simulink model "solarpanel"  (R2023a)
settings: Solver=VariableStepAuto  StartTime=0.0  StopTime=15*3600  RelTol=1e-3
values from neighbouring files (symbols this model uses):
  J = 8.6    [solarpanel.mat]
  Kd = 5    [solarpanel.mat]
  Kf = 0.07    [solarpanel.mat]
  Kg = 2000    [solarpanel.mat]
  Kt = 0.07    [solarpanel.mat]
  L = 1e-05    [solarpanel.mat]
  R = 10    [solarpanel.mat]
libraries: slpidlib x1
settings Model: Creator=brian  LastModifiedBy=brian
settings DataIOCC: ExternalInput=[sunTime sunPosition]  LoadExternalInput=on

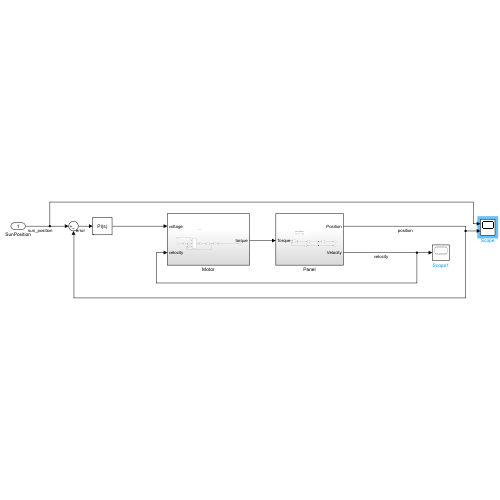
[thumbnail: Simulink's stored preview of the top-level diagram]
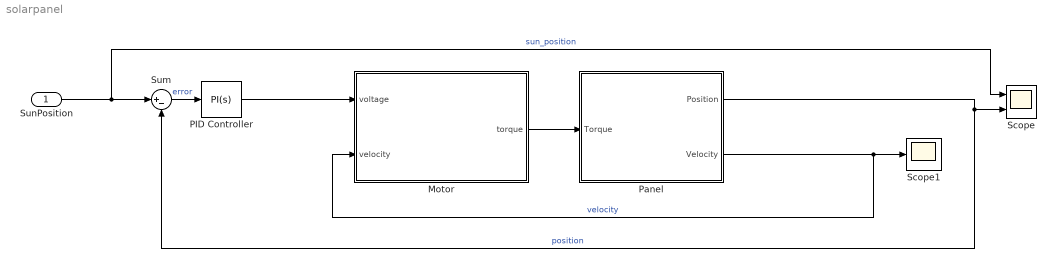
== system solarpanel ==
  SunPosition : Inport
  Motor : Subsystem
  PID Controller : slpidlib/PID Controller  Controller=PI  Form=Parallel  TimeDomain=Continuous-time  UseExternalTs=off  SampleTime=-1  IntegratorMethod=Forward Euler  FilterMethod=Forward Euler  ControllerParametersSource=internal  P=240  I=180  UseKiTs=off  D=0  N=100  UseFilter=on  TunerSelectOption=Transfer Function Based (PID Tuner App)  InitialConditionSource=internal  InitialConditionForIntegrator=0  InitialConditionForFilter=0  DifferentiatorICPrevScaledInput=0  ExternalReset=none  TrackingMode=off  Kt=1  LimitOutput=off  SatLimitsSource=internal  UpperSaturationLimit=inf  LowerSaturationLimit=-inf  LinearizeAsGain=on  AntiWindupMode=none  Kb=1  LimitIntegrator=off  UpperIntegratorSaturationLimit=inf  LowerIntegratorSaturationLimit=-inf  POutMin=[]  POutMax=[]  IOutMin=[]  IOutMax=[]  DOutMin=[]  DOutMax=[]  NOutMin=[]  NOutMax=[]  SumOutMin=[]  SumOutMax=[]  SaturationOutMin=[]  SaturationOutMax=[]  PParamMin=[]  PParamMax=[]  IParamMin=[]  IParamMax=[]  DParamMin=[]  DParamMax=[]  NParamMin=[]  NParamMax=[]  KbParamMin=[]  KbParamMax=[]  KtParamMin=[]  KtParamMax=[]  KbOutMin=[]  KbOutMax=[]  KtOutMin=[]  KtOutMax=[]  IntegratorOutMin=[]  IntegratorOutMax=[]  FilterOutMin=[]  FilterOutMax=[]  SumI1OutMin=[]  SumI1OutMax=[]  SumI2OutMin=[]  SumI2OutMax=[]  SumI3OutMin=[]  SumI3OutMax=[]  SumI4OutMin=[]  SumI4OutMax=[]  SumDOutMin=[]  SumDOutMax=[]  DifferentiatorOutMin=[]  DifferentiatorOutMax=[]  FilterDiffOutCoefMin=[]  FilterDiffOutCoefMax=[]  ReciprocalOutMin=[]  ReciprocalOutMax=[]  SumDenOutMin=[]  SumDenOutMax=[]  SumNumOutMin=[]  SumNumOutMax=[]  DivideOutMin=[]  DivideOutMax=[]  UdiffTsProdOutMin=[]  UdiffTsProdOutMax=[]  NTsProdOutMin=[]  NTsProdOutMax=[]  UintegralTsProdOutMin=[]  UintegralTsProdOutMax=[]  UngainTsProdOutMin=[]  UngainTsProdOutMax=[]  ClampingZeroOutDataTypeStr=Inherit: Inherit via back propagation  ClampingZeroOutMin=[]  ClampingZeroOutMax=[]  FilterDenConstantOutDataTypeStr=Inherit: Inherit via back propagation  FilterDenConstantOutMin=[]  FilterDenConstantOutMax=[]  PCopyOutDataTypeStr=Inherit: Inherit via back propagation  PCopyOutMin=[]  PCopyOutMax=[]  NCopyOutDataTypeStr=Inherit: Inherit via back propagation  NCopyOutMin=[]  NCopyOutMax=[]  IntegratorContinuousStateAttributes=''  IntegratorStateMustResolveToSignalObject=off  IntegratorRTWStateStorageClass=Auto  FilterContinuousStateAttributes=''  FilterStateMustResolveToSignalObject=off  FilterRTWStateStorageClass=Auto  ParallelPVariant=InternalParameters  IdealPVariant=Disabled  IVariant=InternalParameters  DVariant=Disabled  IntegratorVariant=Continuous  SatVariant=Disabled  AWVariant=Passthrough  PCopyVariant=Disabled  TRVariant=Disabled  FdbkBlocksVariant=Forward  IdealPFdbkVariant=Disabled  SatFdbkVariant=Disabled  DerivativeFilterVariant=Disabled  NVariant=Disabled  NCopyVariant=Disabled_SignalSpec  FilterICVariant=Disabled  IntegratorICVariant=InternalICs  ExternalResetVariant=Disabled  TRSumVariant=Passthrough  SumFdbkVariant=Disabled  SumVariant=Sum_PI  TsampFilterVariant=InternalTs  TsampNgainVariant=Passthrough  TsampIntegralVariant=Disabled_SignalSpec  ExternalSaturationOutDataTypeStr=Inherit: Same as second input
  Panel : Subsystem
  Scope : Scope  NumInputPorts=2
  Scope1 : Scope
  Sum : Sum  Inputs=|+-
  wires:
  Panel/1(Position) -> Sum/2, Scope/2  "position"
  Panel/2(Velocity) -> Motor/2(velocity), Scope1/1  "velocity"
  Motor/1(torque) -> Panel/1(Torque)
  PID Controller/1 -> Motor/1(voltage)
  SunPosition/1 -> Scope/1, Sum/1  "sun_position"
  Sum/1 -> PID Controller/1  "error"

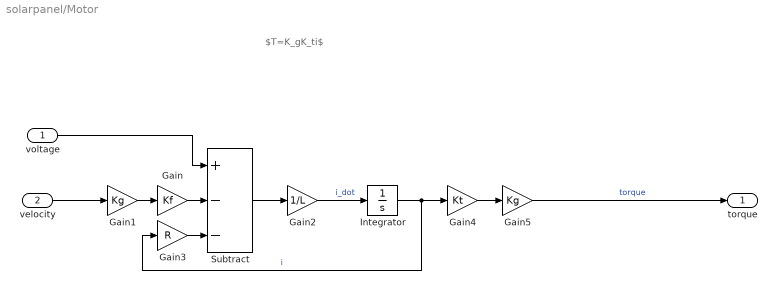
== system solarpanel/Motor ==
  note: $T=K_gK_ti$
  voltage : Inport
  velocity : Inport  Port=2
  Gain : Gain  Gain=Kf
  Gain1 : Gain  Gain=Kg
  Gain2 : Gain  Gain=1/L
  Gain3 : Gain  Gain=R
  Gain4 : Gain  Gain=Kt
  Gain5 : Gain  Gain=Kg
  Integrator : Integrator
  Subtract : Sum  Inputs=+--
  torque : Outport
  wires:
  Gain/1 -> Subtract/2
  Gain4/1 -> Gain5/1
  Integrator/1 -> Gain4/1, Gain3/1  "i"
  Gain2/1 -> Integrator/1  "i_dot"
  velocity/1 -> Gain1/1
  Gain1/1 -> Gain/1
  Gain3/1 -> Subtract/3
  Subtract/1 -> Gain2/1
  Gain5/1 -> torque/1  "torque"
  voltage/1 -> Subtract/1

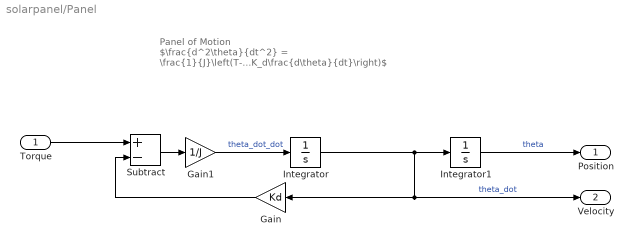
== system solarpanel/Panel ==
  note: Panel of Motion
      | $\frac{d^2\theta}{dt^2} = \frac{1}{J}\left(T-K_d\frac{d\theta}{dt}\right)$
  Torque : Inport
  Gain : Gain  Gain=Kd
  Gain1 : Gain  Gain=1/J
  Integrator : Integrator
  Integrator1 : Integrator
  Subtract : Sum  Inputs=+-
  Position : Outport
  Velocity : Outport  Port=2
  wires:
  Gain1/1 -> Integrator/1  "theta_dot_dot"
  Integrator1/1 -> Position/1  "theta"
  Subtract/1 -> Gain1/1
  Gain/1 -> Subtract/2
  Torque/1 -> Subtract/1
  Integrator/1 -> Velocity/1, Gain/1, Integrator1/1  "theta_dot"
